simulink model "hexa_tilted_quaternion_FxTDiff_ANSFT"  (R2023a)
settings: Solver=ode1  StartTime=0.0  StopTime=60  FixedStep=0.01  RelTol=1e-3
undefined symbols (not defined in the file or in its folder): F, Light, MIL
libraries: sharedtransform x9, dspsrcs4 x9, aerolibutil x7, sharedutil x4, simulink x4, simulink_extras x3, matrix_library x2, robotcorelib x1, aerolibwind2 x1, uavutilslib x1
(part 2 of 2)

== matlab function hexa_tilted_quaternion_FxTDiff_ANSFT/Reference/calculateAttitudeTrajectory ==
  data: qx output; qy output; t input; qz output; w_d output; w_d_dot output
function [qx, qy, qz, w_d, w_d_dot] = fcn(t)

roll = 0.0;
pitch = 0.0;
% yaw = 0;
% w_d = [0; 0; 0];

if t < 5
    % roll = 0;
    % roll_d = 0;
    % pitch = 0;
    yaw = 0;
    w_d = [0; 0; 0];
else
    % roll = 5 * pi / 180 * sin(t - 5);
    % roll_d = 5 * pi / 180 * cos(t - 5);
    yaw = 5 * pi * (t - 5) / 180;
    w_d = [0; 0; 5 * pi / 180];
    % w_d = [0; 0; 0];
    % w_d = [roll_d; 0; 0];
end

qx = [cos(roll/2);
      sin(roll/2);
      0;
      0];

qy = [cos(pitch/2);
      0;
      sin(pitch/2);
      0];

qz = [cos(yaw/2);
      0;
      0;
      sin(yaw/2)];

% w_d = [0; 0; 0];
w_d_dot = [0; 0; 0];

== matlab function hexa_tilted_quaternion_FxTDiff_ANSFT/Controller/Kronecker product4/Kronecker_product ==
  data: q input; r output size=[4 1]; p input
function r = fcn(q, p)

%{
    Function to describe in matrix math the Kronecker product between
    two quaternions
    
    r = p kronecker q
    %}

    len = length(p);

    if len == 3 && length(q) == 4
        p1 = [0; p];
        q0 = q(1);
        q1 = q(2);
        q2 = q(3);
        q3 = q(4);
        
        % skew symmetric matrix
        q_matrix = [q0, -q1, -q2, -q3;
                  q1, q0, -q3, q2;
                  q2, q3, q0, -q1;
                  q3, -q2, q1, q0];
        
        r = q_matrix * p1;

    elseif len == 4
        q0 = q(1);
        q1 = q(2);
        q2 = q(3);
        q3 = q(4);
        
        % skew symmetric matrix
        q_matrix = [q0, -q1, -q2, -q3;
                  q1, q0, -q3, q2;
                  q2, q3, q0, -q1;
                  q3, -q2, q1, q0];
        
        r = q_matrix * p;

    else
        error('Quaternions dimensions do not match')
    end

== matlab function hexa_tilted_quaternion_FxTDiff_ANSFT/Controller/ANSFT parameters ==
  data: xi1 output; xi2 output; lambda1 output; unused input; lambda2 output; alpha output; beta output
function [xi1, xi2, lambda1, lambda2, alpha, beta] = fcn(~)

%% Constantes de la Superficie deslizante
% zeta1 parecido a una ganancia proporcional
xi1 = [2.5; 2.5; 1.5; 1; 1; 1];
%zeta2 parecido a una ganancia derivatida
xi2 = [1.25; 1.25; 2; 0.5; 0.5; 0.5];
% lambda 1 > lambda2
lambda1 = [1.5; 1.5; 1.75; 2; 2; 2];
% 1 < lambda2 < 2
lambda2 = [1.2; 1.2; 1.25; 1.2; 1.2; 1.2];
%% Constantes del control auxiliar
%minimize sigma
alpha = [1.75; 1.75; 0.625; 2.5; 2.5; 1.25];
%aumetnar control, aumentar energía del sistema
beta = [2.5; 2.5; 0.1; 0.05; 0.05; 0.25];

== matlab function hexa_tilted_quaternion_FxTDiff_ANSFT/Controller/Kronecker product6/Kronecker_product ==
  data: q input; r output; p input
function r = fcn(q, p)

%{
    Function to describe in matrix math the Kronecker product between
    two quaternions
    
    r = p kronecker q
    %}

    len = length(p);

    if len == 3
        p1 = [0; p];
        q0 = q(1);
        q1 = q(2);
        q2 = q(3);
        q3 = q(4);
        
        % skew symmetric matrix
        q_matrix = [q0, -q1, -q2, -q3;
                  q1, q0, -q3, q2;
                  q2, q3, q0, -q1;
                  q3, -q2, q1, q0];
        
        r = q_matrix * p1;

    elseif len == 4
        q0 = q(1);
        q1 = q(2);
        q2 = q(3);
        q3 = q(4);
        
        % skew symmetric matrix
        q_matrix = [q0, -q1, -q2, -q3;
                  q1, q0, -q3, q2;
                  q2, q3, q0, -q1;
                  q3, -q2, q1, q0];
        
        r = q_matrix * p;

    else
        error('Quaternions dimensions do not match')
    end

== matlab function hexa_tilted_quaternion_FxTDiff_ANSFT/Controller/Kronecker product7/Kronecker_product ==
  data: q input; r output; p input
function r = fcn(q, p)

%{
    Function to describe in matrix math the Kronecker product between
    two quaternions
    
    r = p kronecker q
    %}

    len = length(p);

    if len == 3
        p1 = [0; p];
        q0 = q(1);
        q1 = q(2);
        q2 = q(3);
        q3 = q(4);
        
        % skew symmetric matrix
        q_matrix = [q0, -q1, -q2, -q3;
                  q1, q0, -q3, q2;
                  q2, q3, q0, -q1;
                  q3, -q2, q1, q0];
        
        r = q_matrix * p1;

    elseif len == 4
        q0 = q(1);
        q1 = q(2);
        q2 = q(3);
        q3 = q(4);
        
        % skew symmetric matrix
        q_matrix = [q0, -q1, -q2, -q3;
                  q1, q0, -q3, q2;
                  q2, q3, q0, -q1;
                  q3, -q2, q1, q0];
        
        r = q_matrix * p;

    else
        error('Quaternions dimensions do not match')
    end

== matlab function hexa_tilted_quaternion_FxTDiff_ANSFT/Fixed-Time Diff/Kronecker product/Kronecker_product ==
  data: q input; r output size=[4 1]; p input
function r = fcn(q, p)

%{
    Function to describe in matrix math the Kronecker product between
    two quaternions
    
    r = p kronecker q
    %}

    len = length(p);

    if len == 3 && length(q) == 4
        p1 = [0; p];
        q0 = q(1);
        q1 = q(2);
        q2 = q(3);
        q3 = q(4);
        
        % skew symmetric matrix
        q_matrix = [q0, -q1, -q2, -q3;
                  q1, q0, -q3, q2;
                  q2, q3, q0, -q1;
                  q3, -q2, q1, q0];
        
        r = q_matrix * p1;

    elseif len == 4
        q0 = q(1);
        q1 = q(2);
        q2 = q(3);
        q3 = q(4);
        
        % skew symmetric matrix
        q_matrix = [q0, -q1, -q2, -q3;
                  q1, q0, -q3, q2;
                  q2, q3, q0, -q1;
                  q3, -q2, q1, q0];
        
        r = q_matrix * p;

    else
        error('Quaternions dimensions do not match')
    end

== matlab function hexa_tilted_quaternion_FxTDiff_ANSFT/Fixed-Time Diff/calculateCvMatrix ==
  data: q input; Cv output
function Cv = fcn(q)

q0 = q(1);
q1 = q(2);
q2 = q(3);
q3 = q(4);

Cv = [q0, -q3, q2;
      q3, q0, -q1;
      -q2, q1, q0] * 0.5;

Cv = inv(Cv);

== matlab function hexa_tilted_quaternion_FxTDiff_ANSFT/Fixed-Time Diff/sgn ==
  data: u input; y output
function y = fcn(u)

if (u >= 0)
    y = 1;
else
    y = -1;
end

== matlab function hexa_tilted_quaternion_FxTDiff_ANSFT/Fixed-Time Diff/Kronecker product1/Kronecker_product ==
  data: q input; r output size=[4 1]; p input
function r = fcn(q, p)

%{
    Function to describe in matrix math the Kronecker product between
    two quaternions
    
    r = p kronecker q
    %}

    len = length(p);

    if len == 3 && length(q) == 4
        p1 = [0; p];
        q0 = q(1);
        q1 = q(2);
        q2 = q(3);
        q3 = q(4);
        
        % skew symmetric matrix
        q_matrix = [q0, -q1, -q2, -q3;
                  q1, q0, -q3, q2;
                  q2, q3, q0, -q1;
                  q3, -q2, q1, q0];
        
        r = q_matrix * p1;

    elseif len == 4
        q0 = q(1);
        q1 = q(2);
        q2 = q(3);
        q3 = q(4);
        
        % skew symmetric matrix
        q_matrix = [q0, -q1, -q2, -q3;
                  q1, q0, -q3, q2;
                  q2, q3, q0, -q1;
                  q3, -q2, q1, q0];
        
        r = q_matrix * p;

    else
        error('Quaternions dimensions do not match')
    end

== matlab function hexa_tilted_quaternion_FxTDiff_ANSFT/Fixed-Time Diff/Kronecker product2/Kronecker_product ==
  data: q input; r output size=[4 1]; p input
function r = fcn(q, p)

%{
    Function to describe in matrix math the Kronecker product between
    two quaternions
    
    r = p kronecker q
    %}

    len = length(p);

    if len == 3 && length(q) == 4
        p1 = [0; p];
        q0 = q(1);
        q1 = q(2);
        q2 = q(3);
        q3 = q(4);
        
        % skew symmetric matrix
        q_matrix = [q0, -q1, -q2, -q3;
                  q1, q0, -q3, q2;
                  q2, q3, q0, -q1;
                  q3, -q2, q1, q0];
        
        r = q_matrix * p1;

    elseif len == 4
        q0 = q(1);
        q1 = q(2);
        q2 = q(3);
        q3 = q(4);
        
        % skew symmetric matrix
        q_matrix = [q0, -q1, -q2, -q3;
                  q1, q0, -q3, q2;
                  q2, q3, q0, -q1;
                  q3, -q2, q1, q0];
        
        r = q_matrix * p;

    else
        error('Quaternions dimensions do not match')
    end

== matlab function hexa_tilted_quaternion_FxTDiff_ANSFT/Fixed-Time Diff/Kronecker product3/Kronecker_product ==
  data: q input; r output size=[4 1]; p input
function r = fcn(q, p)

%{
    Function to describe in matrix math the Kronecker product between
    two quaternions
    
    r = p kronecker q
    %}

    len = length(p);

    if len == 3 && length(q) == 4
        p1 = [0; p];
        q0 = q(1);
        q1 = q(2);
        q2 = q(3);
        q3 = q(4);
        
        % skew symmetric matrix
        q_matrix = [q0, -q1, -q2, -q3;
                  q1, q0, -q3, q2;
                  q2, q3, q0, -q1;
                  q3, -q2, q1, q0];
        
        r = q_matrix * p1;

    elseif len == 4
        q0 = q(1);
        q1 = q(2);
        q2 = q(3);
        q3 = q(4);
        
        % skew symmetric matrix
        q_matrix = [q0, -q1, -q2, -q3;
                  q1, q0, -q3, q2;
                  q2, q3, q0, -q1;
                  q3, -q2, q1, q0];
        
        r = q_matrix * p;

    else
        error('Quaternions dimensions do not match')
    end

== matlab function hexa_tilted_quaternion_FxTDiff_ANSFT/Subsystem/MATLAB Function ==
  data: q input; lnq output size=[3 1]
function lnq = fcn(q)

if length(q) == 4
    q0 = q(1);
    
    q_vec = [q(2); q(3); q(4)];

    if norm(q_vec) == 0
        lnq = [0; 0; 0];
    else
        lnq = (q_vec / (norm(q_vec)) ) * acos(q0);
    end
else
    error('Input must be a vector 4 by 1 (Quaternion)')
end

== matlab function hexa_tilted_quaternion_FxTDiff_ANSFT/Dynamics/Kronecker product/Kronecker_product ==
  data: q input; r output size=[4 1]; p input
function r = fcn(q, p)

%{
    Function to describe in matrix math the Kronecker product between
    two quaternions
    
    r = p kronecker q
    %}

    len = length(p);

    if len == 3 && length(q) == 4
        p1 = [0; p];
        q0 = q(1);
        q1 = q(2);
        q2 = q(3);
        q3 = q(4);
        
        % skew symmetric matrix
        q_matrix = [q0, -q1, -q2, -q3;
                  q1, q0, -q3, q2;
                  q2, q3, q0, -q1;
                  q3, -q2, q1, q0];
        
        r = q_matrix * p1;

    elseif len == 4
        q0 = q(1);
        q1 = q(2);
        q2 = q(3);
        q3 = q(4);
        
        % skew symmetric matrix
        q_matrix = [q0, -q1, -q2, -q3;
                  q1, q0, -q3, q2;
                  q2, q3, q0, -q1;
                  q3, -q2, q1, q0];
        
        r = q_matrix * p;

    else
        error('Quaternions dimensions do not match')
    end

== matlab function hexa_tilted_quaternion_FxTDiff_ANSFT/Dynamics/Constants Functions ==
  data: J output; m output; g output
function [J, m, g] = fcn

m = 1.8; % kg

Jxx =  0.0411; % kg m²
Jyy = 0.0478; % kg m²
Jzz = 0.0599; % kg m²

J = [Jxx, 0, 0;
     0, Jyy, 0;
     0, 0, Jzz];

g = [0; 0; 9.81];

== matlab function hexa_tilted_quaternion_FxTDiff_ANSFT/norm ==
  data: u input; y output
function y = fcn(u)

y = norm(u);

== matlab function hexa_tilted_quaternion_FxTDiff_ANSFT/Dynamics/Kronecker product1/Kronecker_product ==
  data: q input; r output; p input
function r = fcn(q, p)

%{
    Function to describe in matrix math the Kronecker product between
    two quaternions
    
    r = p kronecker q
    %}

    len = length(p);

    if len == 3
        p1 = [0; p];
        q0 = q(1);
        q1 = q(2);
        q2 = q(3);
        q3 = q(4);
        
        % skew symmetric matrix
        q_matrix = [q0, -q1, -q2, -q3;
                  q1, q0, -q3, q2;
                  q2, q3, q0, -q1;
                  q3, -q2, q1, q0];
        
        r = q_matrix * p1;

    elseif len == 4
        q0 = q(1);
        q1 = q(2);
        q2 = q(3);
        q3 = q(4);
        
        % skew symmetric matrix
        q_matrix = [q0, -q1, -q2, -q3;
                  q1, q0, -q3, q2;
                  q2, q3, q0, -q1;
                  q3, -q2, q1, q0];
        
        r = q_matrix * p;

    else
        error('Quaternions dimensions do not match')
    end

== matlab function hexa_tilted_quaternion_FxTDiff_ANSFT/Dynamics/Kronecker product2/Kronecker_product ==
  data: q input; r output; p input
function r = fcn(q, p)

%{
    Function to describe in matrix math the Kronecker product between
    two quaternions
    
    r = p kronecker q
    %}

    len = length(p);

    if len == 3
        p1 = [0; p];
        q0 = q(1);
        q1 = q(2);
        q2 = q(3);
        q3 = q(4);
        
        % skew symmetric matrix
        q_matrix = [q0, -q1, -q2, -q3;
                  q1, q0, -q3, q2;
                  q2, q3, q0, -q1;
                  q3, -q2, q1, q0];
        
        r = q_matrix * p1;

    elseif len == 4
        q0 = q(1);
        q1 = q(2);
        q2 = q(3);
        q3 = q(4);
        
        % skew symmetric matrix
        q_matrix = [q0, -q1, -q2, -q3;
                  q1, q0, -q3, q2;
                  q2, q3, q0, -q1;
                  q3, -q2, q1, q0];
        
        r = q_matrix * p;

    else
        error('Quaternions dimensions do not match')
    end

== matlab function hexa_tilted_quaternion_FxTDiff_ANSFT/Reference/Kronecker product5/Kronecker_product ==
  data: q input; r output size=[4 1]; p input
function r = fcn(q, p)

%{
    Function to describe in matrix math the Kronecker product between
    two quaternions
    
    r = p kronecker q
    %}

    len = length(p);

    if len == 3 && length(q) == 4
        p1 = [0; p];
        q0 = q(1);
        q1 = q(2);
        q2 = q(3);
        q3 = q(4);
        
        % skew symmetric matrix
        q_matrix = [q0, -q1, -q2, -q3;
                  q1, q0, -q3, q2;
                  q2, q3, q0, -q1;
                  q3, -q2, q1, q0];
        
        r = q_matrix * p1;

    elseif len == 4
        q0 = q(1);
        q1 = q(2);
        q2 = q(3);
        q3 = q(4);
        
        % skew symmetric matrix
        q_matrix = [q0, -q1, -q2, -q3;
                  q1, q0, -q3, q2;
                  q2, q3, q0, -q1;
                  q3, -q2, q1, q0];
        
        r = q_matrix * p;

    else
        error('Quaternions dimensions do not match')
    end

== matlab function hexa_tilted_quaternion_FxTDiff_ANSFT/Reference/Helicoidal Trajectory ==
  data: time input; pose_d output; pose_d_dot output; pose_d_ddot output
function [pose_d, pose_d_dot, pose_d_ddot]= fcn(time)

% pos_z = time / 12;
f = 0.15;
arg = f * (time - 5);
r = 2;

% hover for 5 s | include inclination in roll
% 5 metros al menos

if (time < 5)
    pos_x = 0;
    pos_y = 0;
    % roll = 0;
    pos_z = -0.4 * time;
else
    pos_x = -r + r * cos (arg);
    pos_y = r * sin (arg);
    pos_z = -2;
end

% roll = 0;
% yaw = time * 0;

pose_d = [pos_x;
          pos_y;
          pos_z];
          % roll;
          % 0;
          % yaw];

% pos_z_dot = 1 / 12;

% hover for 5 s
if (time < 5)
    pos_x_dot = 0;
    pos_y_dot = 0;
    pos_z_dot = -0.4;
else
    pos_x_dot = - f * r * sin(arg);
    pos_y_dot = f * r * cos(arg);
    pos_z_dot= 0;
end

% yaw_dot = 0;

pose_d_dot = [pos_x_dot;
              pos_y_dot;
              pos_z_dot];
              % 0;
              % 0;
              % yaw_dot];

pos_z_ddot = 0;
% hover for 5 s
if (time < 5)
    pos_x_ddot = 0;
    pos_y_ddot = 0;
else
    pos_x_ddot = - f * f * r * cos(arg);
    pos_y_ddot = - f * f * r * sin(arg);
end

% yaw_ddot = 0;

pose_d_ddot = [pos_x_ddot;
               pos_y_ddot;
               pos_z_ddot];
               % 0;
               % 0;
               % yaw_ddot];

== matlab function hexa_tilted_quaternion_FxTDiff_ANSFT/Reference/Lemniscate Trajectory ==
  data: time input; pose_d output; pose_d_dot output; pose_d_ddot output
function [pose_d, pose_d_dot, pose_d_ddot]= fcn(time)

%% Positions

arg = time / 4;

pos_x = cos(arg) ./ (1 + sin(arg) .* sin(arg));
pos_y = cos(arg) .* sin(arg) ./ (1 + sin(arg) .* sin(arg));
pos_z = sin(arg);

% yaw = time * 0;

pose_d = [pos_x;
          pos_y;
          pos_z];
          % 0;
          % 0;
          % yaw];

%% Velocities

pos_z_dot = 0.25 * cos(arg);
pos_x_dot = - sin(arg)/(4*(sin(arg)^2 + 1)) - (cos(arg)^2*sin(arg))/(2*(sin(arg)^2 + 1)^2);
pos_y_dot = cos(arg)^2/(4*(sin(arg)^2 + 1)) - sin(arg)^2/(4*(sin(arg)^2 + 1)) - (cos(arg)^2*sin(arg)^2)/(2*(sin(arg)^2 + 1)^2);
% yaw_dot = 0;

pose_d_dot = [pos_x_dot;
              pos_y_dot;
              pos_z_dot];
              % 0;
              % 0;
              % yaw_dot];

%% Accelerations

pos_z_ddot = -0.25 * 0.25 * sin(arg);
pos_x_ddot = 0;
pos_y_ddot = 0;
% yaw_ddot = 0;

pose_d_ddot = [pos_x_ddot;
               pos_y_ddot;
               pos_z_ddot];
               % 0;
               % 0;
               % yaw_ddot];

== matlab function hexa_tilted_quaternion_FxTDiff_ANSFT/Controller/calculatePWM ==
  data: omega2 input; pwm output
function pwm = fcn(omega2)

pwm = -1.3121e-09 .* omega2 .* omega2 + 0.00208 .* omega2 + 1107.922;
